simulink model "FilterChain"  (R2025b)
settings: Solver=FixedStepAuto  StartTime=0.0  StopTime=0.1  FixedStep=20e-9  RelTol=1e-3
values from neighbouring files (symbols this model uses):
  cicCompFilt = design(compSpec,'SystemObject',true)    [FilterChainDesign.m]
  dcBlockFilt = designHighpassIIR(      "FilterOrder", dcBlockParams.filterOrder,      "StopbandAttenuation", dcBlockParams.stopbandAtten,      "SystemObject", true,      "DesignMethod", "butter",      "HalfPowerFrequency", dcBlockParams.normalizedBandwidth      )    [DcBlock.m]    (also in FilterChainDesign.m)
  finalFilt = design(finalSpec,'equiripple','SystemObject',true)    [FilterChainDesign.m]
  hbFilt = design(hbSpec,'SystemObject',true)    [FilterChainDesign.m]
  sysClkFreq = 52e6    (= 52000000)    [FilterChainDesign.m]
undefined symbols (not defined in the file or in its folder): cicParams, compParams, hbParams
libraries: dsphdlfiltering2 x5, simulink x1, hdlsllib x1, dsphdlsigops2 x1, dspsrcs4 x1
settings Model: Creator=aidan  LastModifiedBy=aidan
settings OptimizationCC: BlockReduction=off  ConditionallyExecuteInputs=off
settings DebuggingCC: SingleTaskRateTransMsg=error

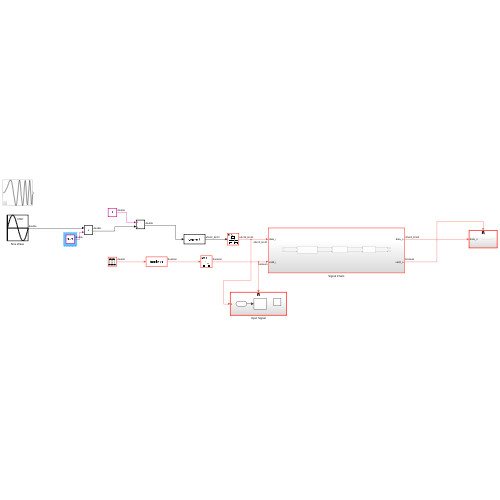
[thumbnail: Simulink's stored preview of the top-level diagram]
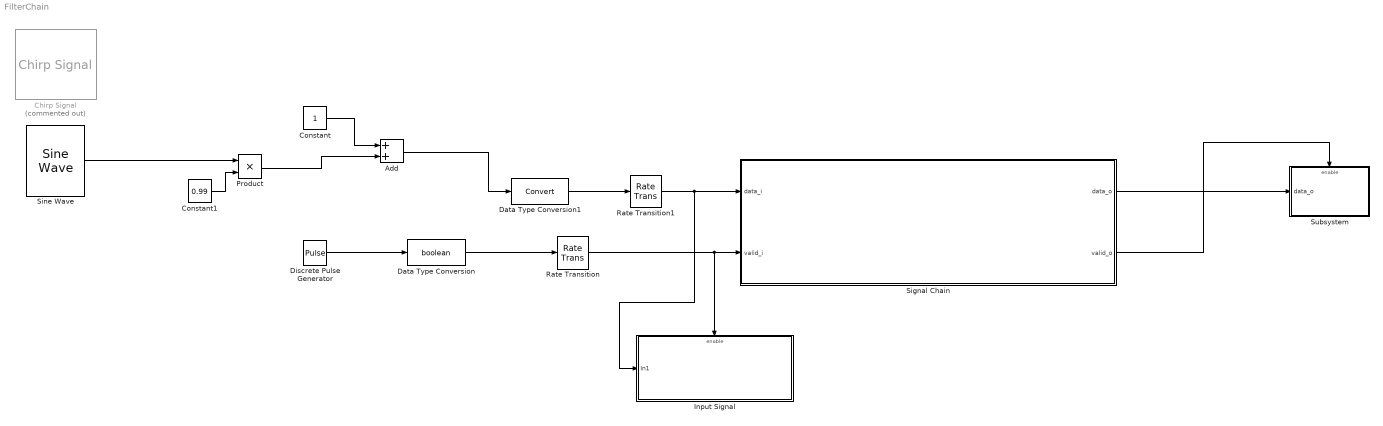
== system FilterChain ==
  Add : Sum
  Chirp Signal : simulink/Sources/Chirp Signal  Commented=on  f1=80000  T=0.1  f2=110000
  Constant : Constant  OutDataTypeStr=double
  Constant1 : Constant  Value=0.99  OutDataTypeStr=double
  Data Type Conversion : DataTypeConversion  OutDataTypeStr=boolean  SaturateOnIntegerOverflow=off  RndMeth=Floor
  Data Type Conversion1 : DataTypeConversion  SaturateOnIntegerOverflow=off  RndMeth=Floor
  Discrete Pulse Generator : DiscretePulseGenerator  Period=50  SampleTime=20e-9
  Input Signal : Subsystem
  Product : Product
  Rate Transition : RateTransition
  Rate Transition1 : RateTransition
  Signal Chain : Subsystem
  Sine Wave : dspsrcs4/Sine Wave  Amplitude=1  Frequency=91400  Phase=1.56  SampleMode=Continuous  OutComplex=Real  CompMethod=Trigonometric fcn  TableSize=Speed  SampleTime=1/1000  SamplesPerFrame=1  ResetState=Restart at time zero  OutputFrames=off  dataType=double  wordLen=16  udDataType=sfix(16)  fracBitsMode=Best precision  numFracBits=15  OutDataTypeStr=double  LastOutDataTypeStr=double
  Subsystem : Subsystem
  wires:
  Discrete Pulse Generator/1 -> Data Type Conversion/1
  Data Type Conversion1/1 -> Rate Transition1/1
  Add/1 -> Data Type Conversion1/1
  Constant/1 -> Add/1
  Data Type Conversion/1 -> Rate Transition/1
  Rate Transition/1 -> Input Signal/Enable, Signal Chain/2(valid_i)
  Signal Chain/2(valid_o) -> Subsystem/Enable
  Constant1/1 -> Product/2
  Product/1 -> Add/2
  Rate Transition1/1 -> Input Signal/1(In1), Signal Chain/1(data_i)
  Sine Wave/1 -> Product/1
  Signal Chain/1(data_o) -> Subsystem/1(data_o)

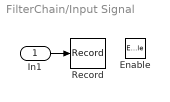
== system FilterChain/Input Signal ==
  In1 : Inport
  Enable : EnablePort
  Record : Record  NumPorts=1.0  FileSettingsInternal="{\"entries\":[{\"content\":{\"excelSettings\":{\"content\":{},\"type\":\"Streamout.ExcelSettings\"},\"parquetSettings\":{\"content\":{},\"type\":\"Streamout.ParquetSettings\"}},\"type\":\"Streamout.FileSettingStorage\",\"uuid\":\"\"}],\"packageUris\":[\"http:\\/\\/schema.mathworks.com\\/mf0\\/streamout_blocks\\/R2020a\"],\"version\":\"1.0\"}"  FrameSettings=0  SignalsInternal="{\"entries\":[{\"content\":{\"signals\":[{\"content\":{\"blockPath\":[],\"dimensions\":[1,1],\"domain\":\"\",\"lineColor\":\"#7e2f8e\",\"lineWidth\":2,\"plots\":[ 1 ],\"port\":1,\"sid\":[\"\"],\"signalID\":1,\"signalName\":\"In1\"},\"type\":\"RecordBlkView.Signal\",\"uuid\":\"\"}]},\"type\":\"RecordBlkView.InputSignals\",\"uuid\":\"\"}],\"packageUris\":[\"http:\\/\\/schema.mathworks.com\\/mf0\\/streamout_blocks\\/R2020a\"],\"version\":\"1.0\"}"  VisualizationBindings="{\"sparklinesplugin\":{\"info\":[{\"bindingParametersList\":[],\"subplotID\":1}]}}"
  wires:
  In1/1 -> Record/1

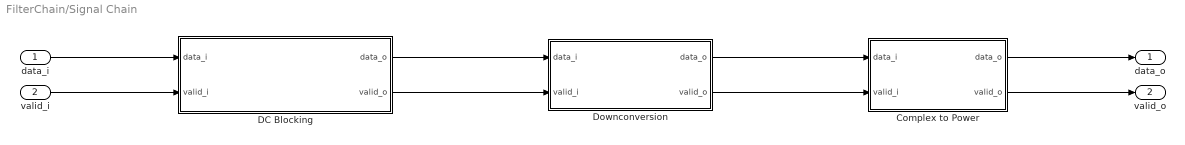
== system FilterChain/Signal Chain ==
  data_i : Inport  OutDataTypeStr=fixdt(0,12,11)
  valid_i : Inport  Port=2  OutDataTypeStr=boolean
  Complex to Power : Subsystem
  DC Blocking : Subsystem
  Downconversion : Subsystem
  data_o : Outport
  valid_o : Outport  Port=2  OutDataTypeStr=boolean
  wires:
  data_i/1 -> DC Blocking/1(data_i)
  valid_i/1 -> DC Blocking/2(valid_i)
  DC Blocking/1(data_o) -> Downconversion/1(data_i)
  DC Blocking/2(valid_o) -> Downconversion/2(valid_i)
  Downconversion/1(data_o) -> Complex to Power/1(data_i)
  Downconversion/2(valid_o) -> Complex to Power/2(valid_i)
  Complex to Power/1(data_o) -> data_o/1
  Complex to Power/2(valid_o) -> valid_o/1

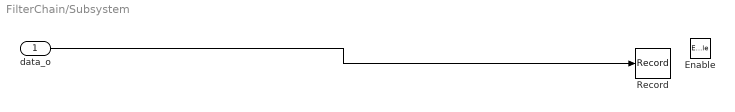
== system FilterChain/Subsystem ==
  data_o : Inport
  Enable : EnablePort
  Record : Record  NumPorts=1.0  FileSettingsInternal="{\"entries\":[{\"content\":{\"excelSettings\":{\"content\":{},\"type\":\"Streamout.ExcelSettings\"},\"parquetSettings\":{\"content\":{},\"type\":\"Streamout.ParquetSettings\"}},\"type\":\"Streamout.FileSettingStorage\",\"uuid\":\"\"}],\"packageUris\":[\"http:\\/\\/schema.mathworks.com\\/mf0\\/streamout_blocks\\/R2020a\"],\"version\":\"1.0\"}"  FrameSettings=0  SignalsInternal="{\"entries\":[{\"content\":{\"signals\":[{\"content\":{\"blockPath\":[],\"dimensions\":[1],\"domain\":\"\",\"lineColor\":\"#4dbeee\",\"lineWidth\":2,\"plots\":[ 1 ],\"port\":1,\"sid\":[\"\"],\"signalID\":1,\"signalName\":\"data_o\"},\"type\":\"RecordBlkView.Signal\",\"uuid\":\"\"}]},\"type\":\"RecordBlkView.InputSignals\",\"uuid\":\"\"}],\"packageUris\":[\"http:\\/\\/schema.mathworks.com\\/mf0\\/streamout_blocks\\/R2020a\"],\"version\":\"1.0\"}"  VisualizationBindings="{\"sparklinesplugin\":{\"info\":[{\"bindingParametersList\":[],\"subplotID\":1}]}}"
  wires:
  data_o/1 -> Record/1

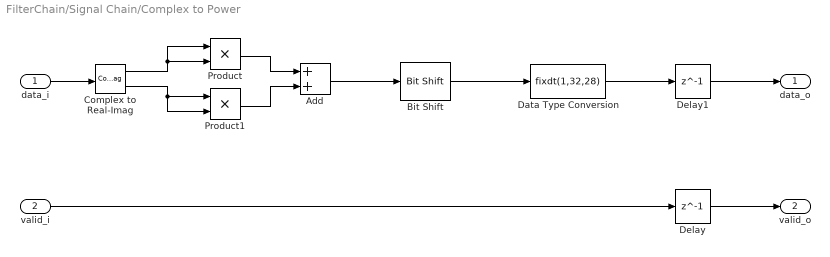
== system FilterChain/Signal Chain/Complex to Power ==
  data_i : Inport
  valid_i : Inport  Port=2
  Add : Sum  OutDataTypeStr=Inherit: Same as accumulator  AccumDataTypeStr=fixdt(1,38,34)
  Bit Shift : hdlsllib/Logic and Bit Operations/Bit Shift  mode=Shift Left Logical  N=1
  Complex to Real-Imag : ComplexToRealImag
  Data Type Conversion : DataTypeConversion  OutDataTypeStr=fixdt(1,32,28)  SaturateOnIntegerOverflow=off  RndMeth=Floor
  Delay : Delay  DelayLength=1  InitialCondition=0
  Delay1 : Delay  DelayLength=1  InitialCondition=0
  Product : Product
  Product1 : Product
  data_o : Outport
  valid_o : Outport  Port=2
  wires:
  valid_i/1 -> Delay/1
  data_i/1 -> Complex to Real-Imag/1
  Complex to Real-Imag/1 -> Product/2, Product/1
  Complex to Real-Imag/2 -> Product1/2, Product1/1
  Product/1 -> Add/1
  Product1/1 -> Add/2
  Add/1 -> Bit Shift/1
  Delay1/1 -> data_o/1
  Delay/1 -> valid_o/1
  Bit Shift/1 -> Data Type Conversion/1
  Data Type Conversion/1 -> Delay1/1

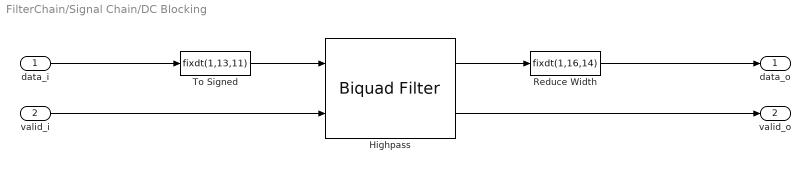
== system FilterChain/Signal Chain/DC Blocking ==
  data_i : Inport  OutDataTypeStr=fixdt(0,12,11)
  valid_i : Inport  Port=2
  Highpass : dsphdlfiltering2/Biquad Filter  Structure=Direct form II transposed  Numerator=dcBlockFilt.Numerator  Denominator=dcBlockFilt.Denominator  ScaleValues=dcBlockFilt.ScaleValues  SimulateUsing=Code generation  roundingMode=Floor  overflowMode=off  NumeratorDataTypeStr=fixdt(1,24,22)  DenominatorDataTypeStr=fixdt(1,24,22)  ScaleValuesDataTypeStr=fixdt(1,24,22)  CoefficientsDataTypeStr=Inherit: Same word length as input  AccumulatorDataTypeStr=fixdt(1,48,40)  OutputDataTypeStr=fixdt(1,48,40)
  Reduce Width : DataTypeConversion  OutDataTypeStr=fixdt(1,16,14)  SaturateOnIntegerOverflow=off  RndMeth=Floor
  To Signed : DataTypeConversion  OutDataTypeStr=fixdt(1,13,11)  SaturateOnIntegerOverflow=off  RndMeth=Floor
  data_o : Outport  OutDataTypeStr=fixdt(1,16,14)
  valid_o : Outport  Port=2
  wires:
  valid_i/1 -> Highpass/2
  Highpass/2 -> valid_o/1
  data_i/1 -> To Signed/1
  To Signed/1 -> Highpass/1
  Highpass/1 -> Reduce Width/1
  Reduce Width/1 -> data_o/1

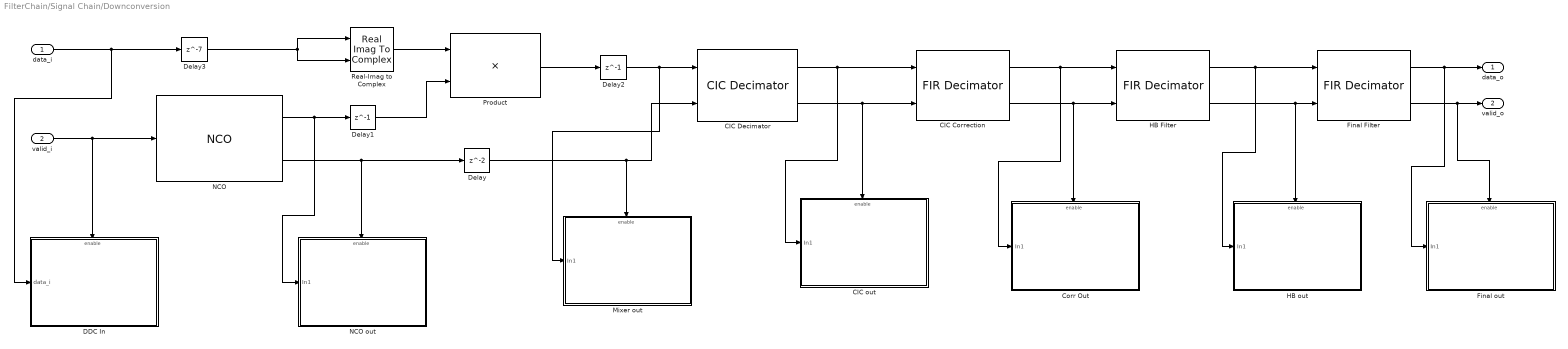
== system FilterChain/Signal Chain/Downconversion ==
  data_i : Inport  OutDataTypeStr=fixdt(1,16,14)
  valid_i : Inport  Port=2  OutDataTypeStr=boolean
  CIC Correction : dsphdlfiltering2/FIR Decimator  NumeratorSource=Property  Numerator=cicCompFilt.Numerator  NumeratorPrototype=[]  FilterStructure=Direct form systolic  DecimationFactor=cicCompFilt.DecimationFactor  NumCycles=ceil(sysClkFreq/cicParams.FsOut)  OptimizeSymmCoeff=on  SimulateUsing=Code generation  roundingMode=Floor  overflowMode=off  CoefficientsDataTypeStr=fixdt(1,24,22)  OutputDataTypeStr=fixdt(1,18,16)  ResetInputPort=off  HDLGlobalReset=on
  CIC Decimator : dsphdlfiltering2/CIC Decimator  DecimationSource=Property  DecimationFactor=cicParams.DecimationFactor  MaxDecimationFactor=2  DifferentialDelay=cicParams.DifferentialDelay  NumSections=cicParams.NumSections  GainCorrection=on  SimulateUsing=Code generation  OutputDataType=Minimum section word lengths  OutputWordLength=18  ResetInputPort=off  HDLGlobalReset=on
  CIC out : Subsystem  TreatAsAtomicUnit=on
  Corr Out : Subsystem  TreatAsAtomicUnit=on
  DDC In : Subsystem  TreatAsAtomicUnit=on
  Delay : Delay  InitialCondition=0
  Delay1 : Delay  DelayLength=1  InitialCondition=0
  Delay2 : Delay  DelayLength=1  InitialCondition=0
  Delay3 : Delay  DelayLength=7  InitialCondition=0
  Final Filter : dsphdlfiltering2/FIR Decimator  NumeratorSource=Property  Numerator=finalFilt.Numerator  NumeratorPrototype=[]  FilterStructure=Direct form systolic  DecimationFactor=finalFilt.DecimationFactor  NumCycles=ceil(sysClkFreq/hbParams.FsOut)  OptimizeSymmCoeff=on  SimulateUsing=Code generation  roundingMode=Floor  overflowMode=off  CoefficientsDataTypeStr=fixdt(1,24,22)  OutputDataTypeStr=fixdt(1,18,17)  ResetInputPort=off  HDLGlobalReset=on
  Final out : Subsystem  TreatAsAtomicUnit=on
  HB Filter : dsphdlfiltering2/FIR Decimator  NumeratorSource=Property  Numerator=hbFilt.Numerator  NumeratorPrototype=[]  FilterStructure=Direct form systolic  DecimationFactor=hbFilt.DecimationFactor  NumCycles=ceil(sysClkFreq/compParams.FsOut)  OptimizeSymmCoeff=on  SimulateUsing=Code generation  roundingMode=Floor  overflowMode=off  CoefficientsDataTypeStr=fixdt(1,24,22)  OutputDataTypeStr=fixdt(1,18,17)  ResetInputPort=off  HDLGlobalReset=on
  HB out : Subsystem  TreatAsAtomicUnit=on
  Mixer out : Subsystem  TreatAsAtomicUnit=on
  NCO : dsphdlsigops2/NCO  PhaseIncrementSource=Property  PhaseIncrement=nco.PhaseInc  PhaseOffsetSource=Property  PhaseOffset=0  DitherSource=Property  NumDitherBits=nco.NumDitherBits  SamplesPerFrame=1  LUTCompress=on  ResetAction=off  Waveform=Complex exponential  PhasePort=off  SimulateUsing=Code generation  AccumulatorWL=nco.AccWL  PhaseQuantization=on  NumQuantizerAccumulatorBits=nco.QuantAccWL  OutputDataType=Binary point scaling  OutputWL=16  OutputFL=14
      settings: LibrarySourceBlock=dsphdlsrcs2/NCO
  NCO out : Subsystem  TreatAsAtomicUnit=on
  Product : Product  InputSameDT=on  OutDataTypeStr=fixdt(1,16,14)
  Real-Imag to Complex : RealImagToComplex
  data_o : Outport
  valid_o : Outport  Port=2
  wires:
  NCO/2 -> NCO out/Enable, Delay/1
  NCO/1 -> NCO out/1(In1), Delay1/1
  Delay1/1 -> Product/2
  Product/1 -> Delay2/1
  Delay2/1 -> Mixer out/1(In1), CIC Decimator/1
  CIC Decimator/2 -> CIC Correction/2, CIC out/Enable
  CIC Decimator/1 -> CIC out/1(In1), CIC Correction/1
  CIC Correction/2 -> Corr Out/Enable, HB Filter/2
  HB Filter/2 -> HB out/Enable, Final Filter/2
  HB Filter/1 -> HB out/1(In1), Final Filter/1
  valid_i/1 -> NCO/1, DDC In/Enable
  Final Filter/1 -> Final out/1(In1), data_o/1
  Final Filter/2 -> Final out/Enable, valid_o/1
  data_i/1 -> DDC In/1(data_i), Delay3/1
  Delay3/1 -> Real-Imag to Complex/1, Real-Imag to Complex/2
  Real-Imag to Complex/1 -> Product/1
  Delay/1 -> CIC Decimator/2, Mixer out/Enable
  CIC Correction/1 -> Corr Out/1(In1), HB Filter/1

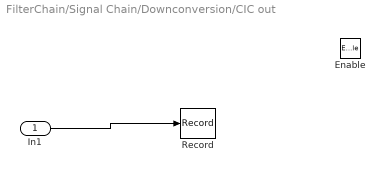
== system FilterChain/Signal Chain/Downconversion/CIC out ==
  In1 : Inport
  Enable : EnablePort
  Record : Record  NumPorts=1.0  FileSettingsInternal="{\"entries\":[{\"content\":{\"excelSettings\":{\"content\":{},\"type\":\"Streamout.ExcelSettings\"},\"parquetSettings\":{\"content\":{},\"type\":\"Streamout.ParquetSettings\"}},\"type\":\"Streamout.FileSettingStorage\",\"uuid\":\"\"}],\"packageUris\":[\"http:\\/\\/schema.mathworks.com\\/mf0\\/streamout_blocks\\/R2020a\"],\"version\":\"1.0\"}"  FrameSettings=0  SignalsInternal="{\"entries\":[{\"content\":{\"signals\":[{\"content\":{\"blockPath\":[],\"dimensions\":[1,1],\"domain\":\"\",\"hasChildren\":true,\"isComplex\":true,\"lineColor\":\"#22b573\",\"lineWidth\":2,\"port\":1,\"sid\":[\"\"],\"signalID\":1,\"signalName\":\"In1\"},\"type\":\"RecordBlkView.Signal\",\"uuid\":\"\"},{\"content\":{\"blockPath\":[],\"dimensions\":[1,1],\"domain\":\"\",\"isComplex\":true,\"lineColor\":\"#64d413\",\"lineWidth\":2,\"parentID\":1,\"plots\":[ 1 ],\"port\":1,\"sid\":[\"\"],\"signalID\":2,\"signalName\":\"In1\"},\"type\":\"RecordBlkView.Signal\",\"uuid\":\"\"},{\"content\":{\"blockPath\":[],\"dimensions\":[1,1],\"domain\":\"\",\"imagPart\":true,\"isComplex\":true,\"lineColor\":\"#d95319\",\"lineWidth\":2,\"parentID\":1,\"port\":1,\"sid\":[\"\"],\"signalID\":3,\"signalName\":\"In1\"},\"type\":\"RecordBlkView.Signal\",\"uuid\":\"\"}]},\"type\":\"RecordBlkView.InputSignals\",\"uuid\":\"\"}],\"packageUris\":[\"http:\\/\\/schema.mathworks.com\\/mf0\\/streamout_blocks\\/R2020a\"],\"version\":\"1.0\"}"  VisualizationBindings="{\"sparklinesplugin\":{\"info\":[{\"bindingParametersList\":[],\"subplotID\":1}]}}"
  wires:
  In1/1 -> Record/1

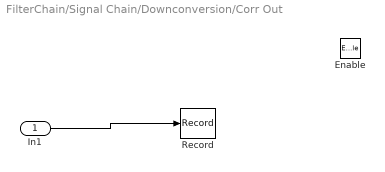
== system FilterChain/Signal Chain/Downconversion/Corr Out ==
  In1 : Inport
  Enable : EnablePort
  Record : Record  NumPorts=1.0  FileSettingsInternal="{\"entries\":[{\"content\":{\"excelSettings\":{\"content\":{},\"type\":\"Streamout.ExcelSettings\"},\"parquetSettings\":{\"content\":{},\"type\":\"Streamout.ParquetSettings\"}},\"type\":\"Streamout.FileSettingStorage\",\"uuid\":\"\"}],\"packageUris\":[\"http:\\/\\/schema.mathworks.com\\/mf0\\/streamout_blocks\\/R2020a\"],\"version\":\"1.0\"}"  FrameSettings=0  SignalsInternal="{\"entries\":[{\"content\":{\"signals\":[{\"content\":{\"blockPath\":[],\"dimensions\":[1,1],\"domain\":\"\",\"hasChildren\":true,\"isComplex\":true,\"lineColor\":\"#edb120\",\"lineWidth\":2,\"port\":1,\"sid\":[\"\"],\"signalID\":1,\"signalName\":\"In1\"},\"type\":\"RecordBlkView.Signal\",\"uuid\":\"\"},{\"content\":{\"blockPath\":[],\"dimensions\":[1,1],\"domain\":\"\",\"isComplex\":true,\"lineColor\":\"#22b573\",\"lineWidth\":2,\"parentID\":1,\"plots\":[ 1 ],\"port\":1,\"sid\":[\"\"],\"signalID\":2,\"signalName\":\"In1\"},\"type\":\"RecordBlkView.Signal\",\"uuid\":\"\"},{\"content\":{\"blockPath\":[],\"dimensions\":[1,1],\"domain\":\"\",\"imagPart\":true,\"isComplex\":true,\"lineColor\":\"#77ac30\",\"lineWidth\":2,\"parentID\":1,\"port\":1,\"sid\":[\"\"],\"signalID\":3,\"signalName\":\"In1\"},\"type\":\"RecordBlkView.Signal\",\"uuid\":\"\"}]},\"type\":\"RecordBlkView.InputSignals\",\"uuid\":\"\"}],\"packageUris\":[\"http:\\/\\/schema.mathworks.com\\/mf0\\/streamout_blocks\\/R2020a\"],\"version\":\"1.0\"}"  VisualizationBindings="{\"sparklinesplugin\":{\"info\":[{\"bindingParametersList\":[],\"subplotID\":1}]}}"
  wires:
  In1/1 -> Record/1

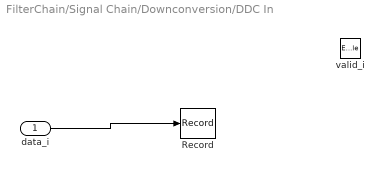
== system FilterChain/Signal Chain/Downconversion/DDC In ==
  data_i : Inport
  valid_i : EnablePort
  Record : Record  NumPorts=1.0  FileSettingsInternal="{\"entries\":[{\"content\":{\"excelSettings\":{\"content\":{},\"type\":\"Streamout.ExcelSettings\"},\"parquetSettings\":{\"content\":{},\"type\":\"Streamout.ParquetSettings\"}},\"type\":\"Streamout.FileSettingStorage\",\"uuid\":\"\"}],\"packageUris\":[\"http:\\/\\/schema.mathworks.com\\/mf0\\/streamout_blocks\\/R2020a\"],\"version\":\"1.0\"}"  FrameSettings=0  SignalsInternal="{\"entries\":[{\"content\":{\"signals\":[{\"content\":{\"blockPath\":[],\"dimensions\":[1,1],\"domain\":\"\",\"lineColor\":\"#77ac30\",\"lineWidth\":2,\"plots\":[ 1 ],\"port\":1,\"sid\":[\"\"],\"signalID\":1,\"signalName\":\"data_i\"},\"type\":\"RecordBlkView.Signal\",\"uuid\":\"\"}]},\"type\":\"RecordBlkView.InputSignals\",\"uuid\":\"\"}],\"packageUris\":[\"http:\\/\\/schema.mathworks.com\\/mf0\\/streamout_blocks\\/R2020a\"],\"version\":\"1.0\"}"  VisualizationBindings="{\"sparklinesplugin\":{\"info\":[{\"bindingParametersList\":[],\"subplotID\":1}]}}"
  wires:
  data_i/1 -> Record/1

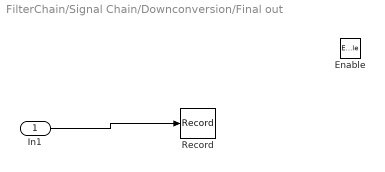
== system FilterChain/Signal Chain/Downconversion/Final out ==
  In1 : Inport
  Enable : EnablePort
  Record : Record  NumPorts=1.0  FileSettingsInternal="{\"entries\":[{\"content\":{\"excelSettings\":{\"content\":{},\"type\":\"Streamout.ExcelSettings\"},\"parquetSettings\":{\"content\":{},\"type\":\"Streamout.ParquetSettings\"}},\"type\":\"Streamout.FileSettingStorage\",\"uuid\":\"\"}],\"packageUris\":[\"http:\\/\\/schema.mathworks.com\\/mf0\\/streamout_blocks\\/R2020a\"],\"version\":\"1.0\"}"  FrameSettings=0  SignalsInternal="{\"entries\":[{\"content\":{\"signals\":[{\"content\":{\"blockPath\":[],\"dimensions\":[1,1],\"domain\":\"\",\"hasChildren\":true,\"isComplex\":true,\"lineColor\":\"#a2142f\",\"lineWidth\":2,\"port\":1,\"sid\":[\"\"],\"signalID\":1,\"signalName\":\"In1\"},\"type\":\"RecordBlkView.Signal\",\"uuid\":\"\"},{\"content\":{\"blockPath\":[],\"dimensions\":[1,1],\"domain\":\"\",\"isComplex\":true,\"lineColor\":\"#7e2f8e\",\"lineWidth\":2,\"parentID\":1,\"plots\":[ 1 ],\"port\":1,\"sid\":[\"\"],\"signalID\":2,\"signalName\":\"In1\"},\"type\":\"RecordBlkView.Signal\",\"uuid\":\"\"},{\"content\":{\"blockPath\":[],\"dimensions\":[1,1],\"domain\":\"\",\"imagPart\":true,\"isComplex\":true,\"lineColor\":\"#ff6929\",\"lineWidth\":2,\"parentID\":1,\"port\":1,\"sid\":[\"\"],\"signalID\":3,\"signalName\":\"In1\"},\"type\":\"RecordBlkView.Signal\",\"uuid\":\"\"}]},\"type\":\"RecordBlkView.InputSignals\",\"uuid\":\"\"}],\"packageUris\":[\"http:\\/\\/schema.mathworks.com\\/mf0\\/streamout_blocks\\/R2020a\"],\"version\":\"1.0\"}"  VisualizationBindings="{\"sparklinesplugin\":{\"info\":[{\"bindingParametersList\":[],\"subplotID\":1}]}}"
  wires:
  In1/1 -> Record/1

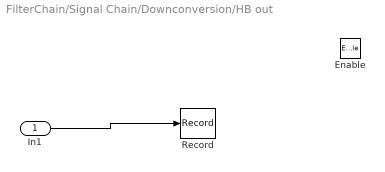
== system FilterChain/Signal Chain/Downconversion/HB out ==
  In1 : Inport
  Enable : EnablePort
  Record : Record  NumPorts=1.0  FileSettingsInternal="{\"entries\":[{\"content\":{\"excelSettings\":{\"content\":{},\"type\":\"Streamout.ExcelSettings\"},\"parquetSettings\":{\"content\":{},\"type\":\"Streamout.ParquetSettings\"}},\"type\":\"Streamout.FileSettingStorage\",\"uuid\":\"\"}],\"packageUris\":[\"http:\\/\\/schema.mathworks.com\\/mf0\\/streamout_blocks\\/R2020a\"],\"version\":\"1.0\"}"  FrameSettings=0  SignalsInternal="{\"entries\":[{\"content\":{\"signals\":[{\"content\":{\"blockPath\":[],\"dimensions\":[1,1],\"domain\":\"\",\"hasChildren\":true,\"isComplex\":true,\"lineColor\":\"#b746ff\",\"lineWidth\":2,\"port\":1,\"sid\":[\"\"],\"signalID\":1,\"signalName\":\"In1\"},\"type\":\"RecordBlkView.Signal\",\"uuid\":\"\"},{\"content\":{\"blockPath\":[],\"dimensions\":[1,1],\"domain\":\"\",\"isComplex\":true,\"lineColor\":\"#a2142f\",\"lineWidth\":2,\"parentID\":1,\"plots\":[ 1 ],\"port\":1,\"sid\":[\"\"],\"signalID\":2,\"signalName\":\"In1\"},\"type\":\"RecordBlkView.Signal\",\"uuid\":\"\"},{\"content\":{\"blockPath\":[],\"dimensions\":[1,1],\"domain\":\"\",\"imagPart\":true,\"isComplex\":true,\"lineColor\":\"#ff13a6\",\"lineWidth\":2,\"parentID\":1,\"port\":1,\"sid\":[\"\"],\"signalID\":3,\"signalName\":\"In1\"},\"type\":\"RecordBlkView.Signal\",\"uuid\":\"\"}]},\"type\":\"RecordBlkView.InputSignals\",\"uuid\":\"\"}],\"packageUris\":[\"http:\\/\\/schema.mathworks.com\\/mf0\\/streamout_blocks\\/R2020a\"],\"version\":\"1.0\"}"  VisualizationBindings="{\"sparklinesplugin\":{\"info\":[{\"bindingParametersList\":[],\"subplotID\":1}]}}"
  wires:
  In1/1 -> Record/1

== system FilterChain/Signal Chain/Downconversion/Mixer out ==
  In1 : Inport
  Enable : EnablePort
  Record : Record  NumPorts=1.0  FileSettingsInternal="{\"entries\":[{\"content\":{\"excelSettings\":{\"content\":{},\"type\":\"Streamout.ExcelSettings\"},\"parquetSettings\":{\"content\":{},\"type\":\"Streamout.ParquetSettings\"}},\"type\":\"Streamout.FileSettingStorage\",\"uuid\":\"\"}],\"packageUris\":[\"http:\\/\\/schema.mathworks.com\\/mf0\\/streamout_blocks\\/R2020a\"],\"version\":\"1.0\"}"  FrameSettings=0  SignalsInternal="{\"entries\":[{\"content\":{\"signals\":[{\"content\":{\"blockPath\":[],\"dimensions\":[1,1],\"domain\":\"\",\"hasChildren\":true,\"isComplex\":true,\"lineColor\":\"#fe330a\",\"lineWidth\":2,\"port\":1,\"sid\":[\"\"],\"signalID\":1,\"signalName\":\"In1\"},\"type\":\"RecordBlkView.Signal\",\"uuid\":\"\"},{\"content\":{\"blockPath\":[],\"dimensions\":[1,1],\"domain\":\"\",\"isComplex\":true,\"lineColor\":\"#b746ff\",\"lineWidth\":2,\"parentID\":1,\"plots\":[ 1 ],\"port\":1,\"sid\":[\"\"],\"signalID\":2,\"signalName\":\"In1\"},\"type\":\"RecordBlkView.Signal\",\"uuid\":\"\"},{\"content\":{\"blockPath\":[],\"dimensions\":[1,1],\"domain\":\"\",\"imagPart\":true,\"isComplex\":true,\"lineColor\":\"#0072bd\",\"lineWidth\":2,\"parentID\":1,\"port\":1,\"sid\":[\"\"],\"signalID\":3,\"signalName\":\"In1\"},\"type\":\"RecordBlkView.Signal\",\"uuid\":\"\"}]},\"type\":\"RecordBlkView.InputSignals\",\"uuid\":\"\"}],\"packageUris\":[\"http:\\/\\/schema.mathworks.com\\/mf0\\/streamout_blocks\\/R2020a\"],\"version\":\"1.0\"}"  VisualizationBindings="{\"sparklinesplugin\":{\"info\":[{\"bindingParametersList\":[],\"subplotID\":1}]}}"
  wires:
  In1/1 -> Record/1

== system FilterChain/Signal Chain/Downconversion/NCO out ==
  In1 : Inport
  Enable : EnablePort
  Record : Record  NumPorts=1.0  FileSettingsInternal="{\"entries\":[{\"content\":{\"excelSettings\":{\"content\":{},\"type\":\"Streamout.ExcelSettings\"},\"parquetSettings\":{\"content\":{},\"type\":\"Streamout.ParquetSettings\"}},\"type\":\"Streamout.FileSettingStorage\",\"uuid\":\"\"}],\"packageUris\":[\"http:\\/\\/schema.mathworks.com\\/mf0\\/streamout_blocks\\/R2020a\"],\"version\":\"1.0\"}"  FrameSettings=0  SignalsInternal="{\"entries\":[{\"content\":{\"signals\":[{\"content\":{\"blockPath\":[],\"dimensions\":[1,1],\"domain\":\"\",\"hasChildren\":true,\"isComplex\":true,\"lineColor\":\"#d95319\",\"lineWidth\":2,\"port\":1,\"sid\":[\"\"],\"signalID\":1,\"signalName\":\"In1\"},\"type\":\"RecordBlkView.Signal\",\"uuid\":\"\"},{\"content\":{\"blockPath\":[],\"dimensions\":[1,1],\"domain\":\"\",\"isComplex\":true,\"lineColor\":\"#ff13a6\",\"lineWidth\":2,\"parentID\":1,\"plots\":[ 1 ],\"port\":1,\"sid\":[\"\"],\"signalID\":2,\"signalName\":\"In1\"},\"type\":\"RecordBlkView.Signal\",\"uuid\":\"\"},{\"content\":{\"blockPath\":[],\"dimensions\":[1,1],\"domain\":\"\",\"imagPart\":true,\"isComplex\":true,\"lineColor\":\"#7e2f8e\",\"lineWidth\":2,\"parentID\":1,\"port\":1,\"sid\":[\"\"],\"signalID\":3,\"signalName\":\"In1\"},\"type\":\"RecordBlkView.Signal\",\"uuid\":\"\"}]},\"type\":\"RecordBlkView.InputSignals\",\"uuid\":\"\"}],\"packageUris\":[\"http:\\/\\/schema.mathworks.com\\/mf0\\/streamout_blocks\\/R2020a\"],\"version\":\"1.0\"}"  VisualizationBindings="{\"sparklinesplugin\":{\"info\":[{\"bindingParametersList\":[],\"subplotID\":1}]}}"
  wires:
  In1/1 -> Record/1
